simulink model "visual_line_follower_ppo_residual"  (R2026a)
settings: Solver=FixedStepDiscrete  StopTime=50  FixedStep=MJ_StepTime  EnableMultiTasking=on
InitFcn:
  | run(fullfile(fileparts(get_param(bdroot,"FileName")),"runtime","configure_turtlebot3_visual_line_follower_paths.m"));
model workspace (MAT data in the model file):
  BaseLinearSpeed = 20
  BaseSpeedScale = 0.03
  Kd_Line = 0.35
  Ki_Line = 0
  Kp_Line = 5
  LocalPath_CurvatureGain = 0.04
  LocalPath_HeadingGain = 0.35
  LocalPath_LateralGain = 0.6
  LocalPath_LookaheadDistance = 0.2
  LocalPath_NumPoints = 30
  LocalPath_ROIFraction = 0.5
  MJ_StepTime = 0.002
  MJ_TargetLateralPosition = 0
  MaxAngularSpeed = 1.5
  MaxWheelSpeed = 25
  N_Line = 20
  OriginBot_ErrorScale = 500
  OriginBot_MaxSaturation = 0.3
  OriginBot_MinBrightness = 70
  OriginBot_MinPixels = 30
  OriginBot_ROIHeight = 45
  OriginBot_ROIStartFraction = 0.72
  PPO_Done_Steps = 100
  PPO_MaxDeltaOmega = 1
  PPO_P_Lost = 10
  PPO_Q = 1
  PPO_R = 0.1
  SteeringSign = -1
  TB3_WheelRadius = 0.033
  TB3_WheelSeparation = 0.16
  Ts_Control = 0.05
  Ts_Stop = 10
  Ts_Vision = 0.05
  TurtleBot3MuJoCoMap = "track_hard"
  TurtleBot3MuJoCoScene = ""
undefined symbols (not defined in the file): originbot_line_follower_debug_frame, originbot_sliding_window_path_generator
libraries: mjLib x1, slpidlib x1, rllib x1
settings Model: ExtModeTrigDuration=10000  Creator=HP  LastModifiedBy=HP
settings SolverCC: PositivePriorityOrder=on
settings ConfigComp: CovMetricSettings=dswe

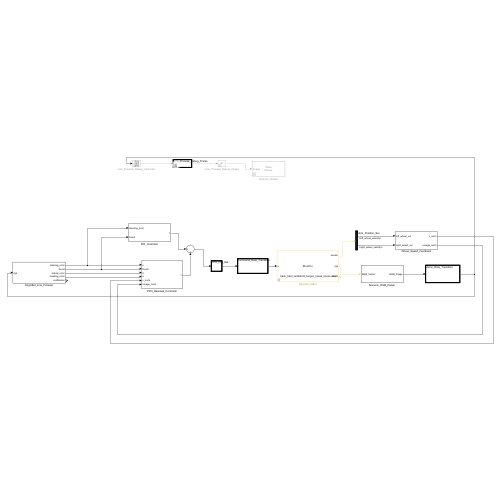
[thumbnail: Simulink's stored preview of the top-level diagram]
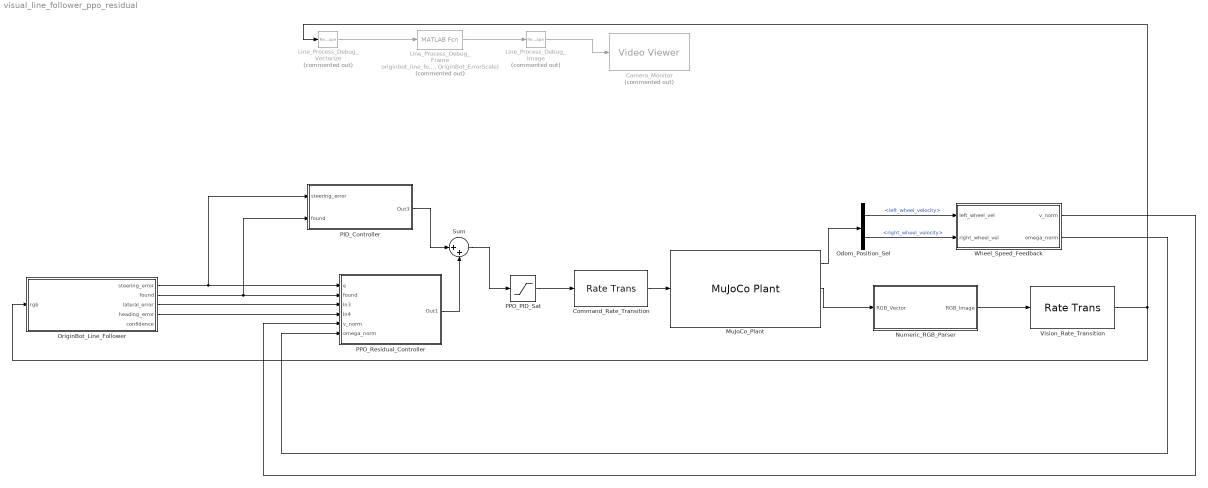
== system visual_line_follower_ppo_residual ==
  Camera_Monitor : VideoViewer  Commented=on  FigPos=[498 692 990 438]
  Command_Rate_Transition : RateTransition  OutPortSampleTime=MJ_StepTime
  Line_Process_Debug_Frame : MATLABFcn  Commented=on  MATLABFcn=originbot_line_follower_debug_frame(u, LocalPath_ROIFraction, LocalPath_NumPoints, OriginBot_MinBrightness, OriginBot_MaxSaturation, OriginBot_MinPixels, OriginBot_ErrorScale)
  Line_Process_Debug_Image : Reshape  Commented=on  OutputDimensionality=Customize  OutputDimensions=[480,640,3]
  Line_Process_Debug_Vectorize : Reshape  Commented=on  OutputDimensionality=Column vector (2-D)
  MuJoCo_Plant : mjLib/MuJoCo Plant  controlBus=[]  sensorBus=mj_bus_sensor_7979902499018342666  controlLength=[]  sensorLength=[]  rgbLength=[]  depthLength=[]  sampleTime=0.002  xmlFileRel=/media/kevin/ding/final_project/Sheffield/for_getting_started/src/simple_camera_pid/matlab/../../../model/mujoco/turtlebot3/track_hard_turtlebot3_burger_visual_scene.xml  xmlFile=/media/kevin/ding/final_project/Sheffield/for_getting_started/src/simple_camera_pid/matlab/../../../model/mujoco/turtlebot3/track_hard_turtlebot3_burger_visual_scene.xml  renderingType=None  vsync=on  visualFPS=60  zoomLevel=1  znear=0.062275  zfar=311.3772  cameraSampleTime=Ts_Vision  rgbOutOption=on  depthOutOption=off  controlInterfaceType=Vector
      settings: SourceProductName=MuJoCo Simulator
  Numeric_RGB_Parser : Subsystem
  Odom_Position_Sel : BusSelector  OutputSignals=left_wheel_velocity,right_wheel_velocity
  OriginBot_Line_Follower : Subsystem
  PID_Controller : Subsystem
  PPO_PID_Sat : Saturate  UpperLimit=[MaxWheelSpeed; MaxWheelSpeed]  LowerLimit=-[MaxWheelSpeed; MaxWheelSpeed]
  PPO_Residual_Controller : Subsystem
  Sum : Sum  Inputs=|++
  Vision_Rate_Transition : RateTransition  OutPortSampleTime=Ts_Vision
  Wheel_Speed_Feedback : Subsystem
  wires:
  Wheel_Speed_Feedback/2(omega_norm) -> PPO_Residual_Controller/6(omega_norm)
  Wheel_Speed_Feedback/1(v_norm) -> PPO_Residual_Controller/5(v_norm)
  Odom_Position_Sel/2 -> Wheel_Speed_Feedback/2(right_wheel_vel)  "<right_wheel_velocity>"
  Odom_Position_Sel/1 -> Wheel_Speed_Feedback/1(left_wheel_vel)  "<left_wheel_velocity>"
  Line_Process_Debug_Frame/1 -> Line_Process_Debug_Image/1
  Vision_Rate_Transition/1 -> OriginBot_Line_Follower/1(rgb), Line_Process_Debug_Vectorize/1
  Line_Process_Debug_Vectorize/1 -> Line_Process_Debug_Frame/1
  MuJoCo_Plant/2 -> Numeric_RGB_Parser/1(RGB_Vector)
  OriginBot_Line_Follower/2(found) -> PID_Controller/2(found), PPO_Residual_Controller/2(found)
  OriginBot_Line_Follower/1(steering_error) -> PID_Controller/1(steering_error), PPO_Residual_Controller/1(e)
  Command_Rate_Transition/1 -> MuJoCo_Plant/1
  Line_Process_Debug_Image/1 -> Camera_Monitor/1
  Numeric_RGB_Parser/1(RGB_Image) -> Vision_Rate_Transition/1
  OriginBot_Line_Follower/3(lateral_error) -> PPO_Residual_Controller/3(In3)
  OriginBot_Line_Follower/4(heading_error) -> PPO_Residual_Controller/4(In4)
  PID_Controller/1(Out3) -> Sum/1
  PPO_Residual_Controller/1(Out1) -> Sum/2
  Sum/1 -> PPO_PID_Sat/1
  PPO_PID_Sat/1 -> Command_Rate_Transition/1
  MuJoCo_Plant/1 -> Odom_Position_Sel/1

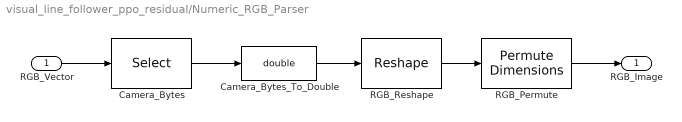
== system visual_line_follower_ppo_residual/Numeric_RGB_Parser ==
  RGB_Vector : Inport
  Camera_Bytes : Selector  InputPortWidth=921601  IndexOptions=Index vector (dialog)  Indices=1:921600  OutputSizes=1
  Camera_Bytes_To_Double : DataTypeConversion  OutDataTypeStr=double
  RGB_Permute : PermuteDimensions  Order=[3 2 1]
  RGB_Reshape : Reshape  OutputDimensionality=Customize  OutputDimensions=[3,640,480]
  RGB_Image : Outport
  wires:
  Camera_Bytes_To_Double/1 -> RGB_Reshape/1
  RGB_Permute/1 -> RGB_Image/1
  RGB_Reshape/1 -> RGB_Permute/1
  Camera_Bytes/1 -> Camera_Bytes_To_Double/1
  RGB_Vector/1 -> Camera_Bytes/1

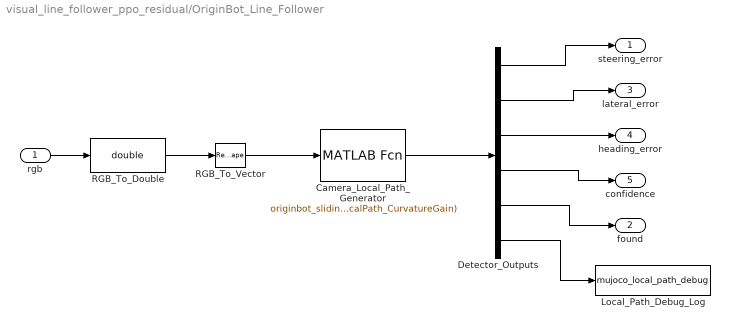
== system visual_line_follower_ppo_residual/OriginBot_Line_Follower ==
  rgb : Inport
  Camera_Local_Path_Generator : MATLABFcn  MATLABFcn=originbot_sliding_window_path_generator(u, LocalPath_ROIFraction, LocalPath_NumPoints, OriginBot_MinBrightness, OriginBot_MaxSaturation, OriginBot_MinPixels, OriginBot_ErrorScale, LocalPath_LookaheadDistance, LocalPath_LateralGain, LocalPath_HeadingGain, LocalPath_CurvatureGain)  OutputDimensions=72  OutputSignalType=real  SampleTime=Ts_Vision
  Detector_Outputs : Demux  Outputs=[1 1 1 1 1 67]
  Local_Path_Debug_Log : ToWorkspace  VariableName=mujoco_local_path_debug  SaveFormat=Timeseries  SampleTime=-1
  RGB_To_Double : DataTypeConversion  OutDataTypeStr=double
  RGB_To_Vector : Reshape  OutputDimensionality=Column vector (2-D)
  steering_error : Outport
  found : Outport  Port=2
  lateral_error : Outport  Port=3
  heading_error : Outport  Port=4
  confidence : Outport  Port=5
  wires:
  Detector_Outputs/2 -> lateral_error/1
  rgb/1 -> RGB_To_Double/1
  RGB_To_Double/1 -> RGB_To_Vector/1
  RGB_To_Vector/1 -> Camera_Local_Path_Generator/1
  Detector_Outputs/4 -> confidence/1
  Camera_Local_Path_Generator/1 -> Detector_Outputs/1
  Detector_Outputs/1 -> steering_error/1
  Detector_Outputs/3 -> heading_error/1
  Detector_Outputs/5 -> found/1
  Detector_Outputs/6 -> Local_Path_Debug_Log/1

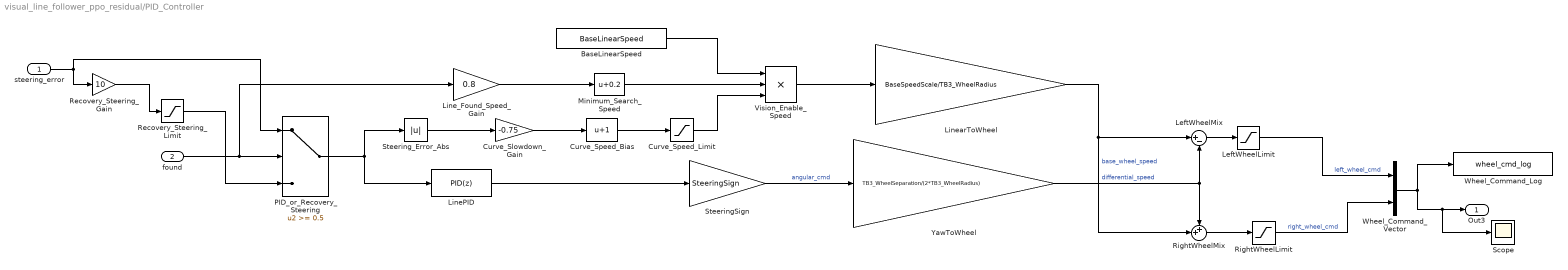
== system visual_line_follower_ppo_residual/PID_Controller ==
  steering_error : Inport
  found : Inport  Port=2
  BaseLinearSpeed : Constant  Value=BaseLinearSpeed
  Curve_Slowdown_Gain : Gain  Gain=-0.75
  Curve_Speed_Bias : Bias  Bias=1
  Curve_Speed_Limit : Saturate  UpperLimit=1  LowerLimit=0.25
  LeftWheelLimit : Saturate  UpperLimit=MaxWheelSpeed  LowerLimit=-MaxWheelSpeed
  LeftWheelMix : Sum  Inputs=|+-
  LinePID : slpidlib/PID Controller  Controller=PID  Form=Parallel  TimeDomain=Discrete-time  UseExternalTs=off  SampleTime=Ts_Control  IntegratorMethod=Backward Euler  FilterMethod=Trapezoidal  ControllerParametersSource=internal  P=Kp_Line  I=Ki_Line  UseKiTs=off  D=Kd_Line  UseExternalDerivativeSource=off  N=N_Line  UseFilter=on  TunerSelectOption=Transfer Function Based (PID Tuner App)  InitialConditionSource=internal  InitialConditionForIntegrator=0  InitialConditionForFilter=0  DifferentiatorICPrevScaledInput=0  ExternalReset=none  TrackingMode=off  Kt=1  LimitOutput=on  SatLimitsSource=internal  UpperSaturationLimit=MaxAngularSpeed  LowerSaturationLimit=-MaxAngularSpeed  LinearizeAsGain=off  AntiWindupMode=back-calculation  Kb=1  LimitIntegrator=off  UpperIntegratorSaturationLimit=inf  LowerIntegratorSaturationLimit=-inf  POutMin=[]  POutMax=[]  IOutMin=[]  IOutMax=[]  DOutMin=[]  DOutMax=[]  NOutMin=[]  NOutMax=[]  SumOutMin=[]  SumOutMax=[]  SaturationOutMin=[]  SaturationOutMax=[]  PParamMin=[]  PParamMax=[]  IParamMin=[]  IParamMax=[]  DParamMin=[]  DParamMax=[]  NParamMin=[]  NParamMax=[]  KbParamMin=[]  KbParamMax=[]  KtParamMin=[]  KtParamMax=[]  KbOutMin=[]  KbOutMax=[]  KtOutMin=[]  KtOutMax=[]  IntegratorOutMin=[]  IntegratorOutMax=[]  FilterOutMin=[]  FilterOutMax=[]  SumI1OutMin=[]  SumI1OutMax=[]  SumI2OutMin=[]  SumI2OutMax=[]  SumI3OutMin=[]  SumI3OutMax=[]  SumI4OutMin=[]  SumI4OutMax=[]  SumDOutMin=[]  SumDOutMax=[]  DifferentiatorOutMin=[]  DifferentiatorOutMax=[]  FilterDiffOutCoefMin=[]  FilterDiffOutCoefMax=[]  ReciprocalOutMin=[]  ReciprocalOutMax=[]  SumDenOutMin=[]  SumDenOutMax=[]  SumNumOutMin=[]  SumNumOutMax=[]  DivideOutMin=[]  DivideOutMax=[]  UdiffTsProdOutMin=[]  UdiffTsProdOutMax=[]  NTsProdOutMin=[]  NTsProdOutMax=[]  UintegralTsProdOutMin=[]  UintegralTsProdOutMax=[]  UngainTsProdOutMin=[]  UngainTsProdOutMax=[]  ClampingZeroOutDataTypeStr=Inherit: Inherit via back propagation  ClampingZeroOutMin=[]  ClampingZeroOutMax=[]  FilterDenConstantOutDataTypeStr=Inherit: Inherit via back propagation  FilterDenConstantOutMin=[]  FilterDenConstantOutMax=[]  PCopyOutDataTypeStr=Inherit: Inherit via back propagation  PCopyOutMin=[]  PCopyOutMax=[]  NCopyOutDataTypeStr=Inherit: Inherit via back propagation  NCopyOutMin=[]  NCopyOutMax=[]  IntegratorContinuousStateAttributes=''  IntegratorStateMustResolveToSignalObject=off  IntegratorRTWStateStorageClass=Auto  FilterContinuousStateAttributes=''  FilterStateMustResolveToSignalObject=off  FilterRTWStateStorageClass=Auto  ParallelPVariant=InternalParameters  IdealPVariant=Disabled  IVariant=InternalParameters  DVariant=InternalParameters  IntegratorVariant=Discrete  SatVariant=Enabled  AWVariant=BackCalculation  PCopyVariant=Disabled  TRVariant=Disabled  FdbkBlocksVariant=Feedback  IdealPFdbkVariant=Passthrough  SatFdbkVariant=Enabled  DerivativeFilterVariant=TrapezoidalFilter  NVariant=InternalParameters  NCopyVariant=InternalParameters  FilterICVariant=InternalICsFilter  IntegratorICVariant=InternalICs  ExternalResetVariant=Disabled  TRSumVariant=Passthrough  SumFdbkVariant=Enabled  SumVariant=Sum_PID  TsampFilterVariant=InternalTs  TsampNgainVariant=Passthrough  TsampIntegralVariant=Disabled_SignalSpec  ExternalSaturationOutDataTypeStr=Inherit: Same as second input  DerivativeSourceVariant=ErrorSignal  PreIntVariant=InternalPreInt
      settings: LibrarySourceBlock=hdlsllib/Discrete/Discrete PID Controller
  Line_Found_Speed_Gain : Gain  Gain=0.8
  LinearToWheel : Gain  Gain=BaseSpeedScale/TB3_WheelRadius
  Minimum_Search_Speed : Bias  Bias=0.2
  PID_or_Recovery_Steering : Switch  Threshold=0.5
  Recovery_Steering_Gain : Gain  Gain=10
  Recovery_Steering_Limit : Saturate  UpperLimit=0.45  LowerLimit=-0.45
  RightWheelLimit : Saturate  UpperLimit=MaxWheelSpeed  LowerLimit=-MaxWheelSpeed
  RightWheelMix : Sum  Inputs=++|
  Scope : Scope
  SteeringSign : Gain  Gain=SteeringSign
  Steering_Error_Abs : Abs
  Vision_Enable_Speed : Product  Inputs=***
  Wheel_Command_Log : ToWorkspace  VariableName=wheel_cmd_log  SaveFormat=Structure With Time
  Wheel_Command_Vector : Mux  Inputs=2
  YawToWheel : Gain  Gain=TB3_WheelSeparation/(2*TB3_WheelRadius)
  Out3 : Outport
  wires:
  LeftWheelLimit/1 -> Wheel_Command_Vector/1  "left_wheel_cmd"
  steering_error/1 -> Recovery_Steering_Gain/1, PID_or_Recovery_Steering/1
  Minimum_Search_Speed/1 -> Vision_Enable_Speed/2
  found/1 -> Line_Found_Speed_Gain/1, PID_or_Recovery_Steering/2
  PID_or_Recovery_Steering/1 -> Steering_Error_Abs/1, LinePID/1
  Recovery_Steering_Gain/1 -> Recovery_Steering_Limit/1
  Recovery_Steering_Limit/1 -> PID_or_Recovery_Steering/3
  Line_Found_Speed_Gain/1 -> Minimum_Search_Speed/1
  Steering_Error_Abs/1 -> Curve_Slowdown_Gain/1
  Curve_Slowdown_Gain/1 -> Curve_Speed_Bias/1
  Curve_Speed_Bias/1 -> Curve_Speed_Limit/1
  LinePID/1 -> SteeringSign/1
  BaseLinearSpeed/1 -> Vision_Enable_Speed/1
  Curve_Speed_Limit/1 -> Vision_Enable_Speed/3
  Vision_Enable_Speed/1 -> LinearToWheel/1
  SteeringSign/1 -> YawToWheel/1  "angular_cmd"
  LinearToWheel/1 -> LeftWheelMix/1, RightWheelMix/2  "base_wheel_speed"
  YawToWheel/1 -> RightWheelMix/1, LeftWheelMix/2  "differential_speed"
  LeftWheelMix/1 -> LeftWheelLimit/1
  RightWheelMix/1 -> RightWheelLimit/1
  RightWheelLimit/1 -> Wheel_Command_Vector/2  "right_wheel_cmd"
  Wheel_Command_Vector/1 -> Scope/1, Out3/1, Wheel_Command_Log/1

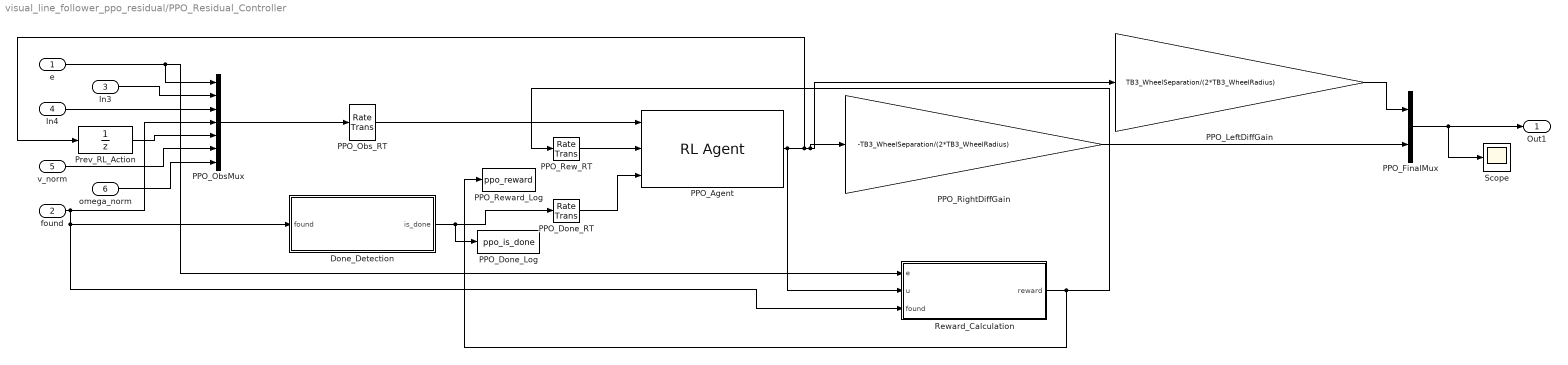
== system visual_line_follower_ppo_residual/PPO_Residual_Controller ==
  e : Inport
  found : Inport  Port=2
  In3 : Inport  Port=3
  In4 : Inport  Port=4
  v_norm : Inport  Port=5
  omega_norm : Inport  Port=6
  Done_Detection : Subsystem
  PPO_Agent : rllib/RL Agent  Agent=agent  ExternalActionAsInput=off  ProvideLastAction=off  ProvideCumRwd=off  TreatAsDirectFeedthrough=on  UseStrictObservationDataTypes=off
  PPO_Done_Log : ToWorkspace  VariableName=ppo_is_done  SaveFormat=Timeseries  SampleTime=-1
  PPO_Done_RT : RateTransition  Integrity=off  Deterministic=off
  PPO_FinalMux : Mux  Inputs=2
  PPO_LeftDiffGain : Gain  Gain=TB3_WheelSeparation/(2*TB3_WheelRadius)
  PPO_ObsMux : Mux  Inputs=7
  PPO_Obs_RT : RateTransition  Integrity=off  Deterministic=off
  PPO_Rew_RT : RateTransition  Integrity=off  Deterministic=off
  PPO_Reward_Log : ToWorkspace  VariableName=ppo_reward  SaveFormat=Timeseries  SampleTime=-1
  PPO_RightDiffGain : Gain  Gain=-TB3_WheelSeparation/(2*TB3_WheelRadius)
  Prev_RL_Action : UnitDelay  SampleTime=Ts_Control
  Reward_Calculation : Subsystem
  Scope : Scope
      settings: ActiveDisplayYMinimum=-1  ActiveDisplayYMaximum=1
  Out1 : Outport
  wires:
  omega_norm/1 -> PPO_ObsMux/7
  v_norm/1 -> PPO_ObsMux/6
  Done_Detection/1(is_done) -> PPO_Done_RT/1, PPO_Done_Log/1
  Reward_Calculation/1(reward) -> PPO_Reward_Log/1, PPO_Rew_RT/1
  PPO_FinalMux/1 -> Out1/1, Scope/1
  PPO_RightDiffGain/1 -> PPO_FinalMux/2
  PPO_LeftDiffGain/1 -> PPO_FinalMux/1
  PPO_ObsMux/1 -> PPO_Obs_RT/1
  Prev_RL_Action/1 -> PPO_ObsMux/5
  In4/1 -> PPO_ObsMux/3
  In3/1 -> PPO_ObsMux/2
  PPO_Agent/1 -> PPO_LeftDiffGain/1, PPO_RightDiffGain/1, Prev_RL_Action/1, Reward_Calculation/2(u)
  PPO_Obs_RT/1 -> PPO_Agent/1
  PPO_Done_RT/1 -> PPO_Agent/3
  PPO_Rew_RT/1 -> PPO_Agent/2
  found/1 -> Reward_Calculation/3(found), Done_Detection/1(found), PPO_ObsMux/4
  e/1 -> Reward_Calculation/1(e), PPO_ObsMux/1

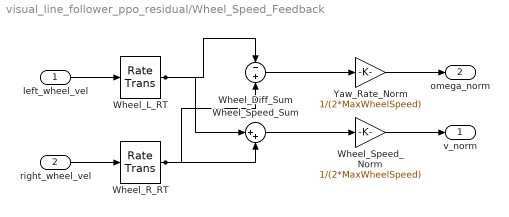
== system visual_line_follower_ppo_residual/Wheel_Speed_Feedback ==
  left_wheel_vel : Inport
  right_wheel_vel : Inport  Port=2
  Wheel_Diff_Sum : Sum  Inputs=-+
  Wheel_L_RT : RateTransition  OutPortSampleTime=Ts_Control
  Wheel_R_RT : RateTransition  OutPortSampleTime=Ts_Control
  Wheel_Speed_Norm : Gain  Gain=1/(2*MaxWheelSpeed)
  Wheel_Speed_Sum : Sum  Inputs=|++
  Yaw_Rate_Norm : Gain  Gain=1/(2*MaxWheelSpeed)
  v_norm : Outport
  omega_norm : Outport  Port=2
  wires:
  Yaw_Rate_Norm/1 -> omega_norm/1
  Wheel_Speed_Norm/1 -> v_norm/1
  Wheel_Diff_Sum/1 -> Yaw_Rate_Norm/1
  Wheel_Speed_Sum/1 -> Wheel_Speed_Norm/1
  Wheel_R_RT/1 -> Wheel_Speed_Sum/2, Wheel_Diff_Sum/2
  Wheel_L_RT/1 -> Wheel_Speed_Sum/1, Wheel_Diff_Sum/1
  right_wheel_vel/1 -> Wheel_R_RT/1
  left_wheel_vel/1 -> Wheel_L_RT/1

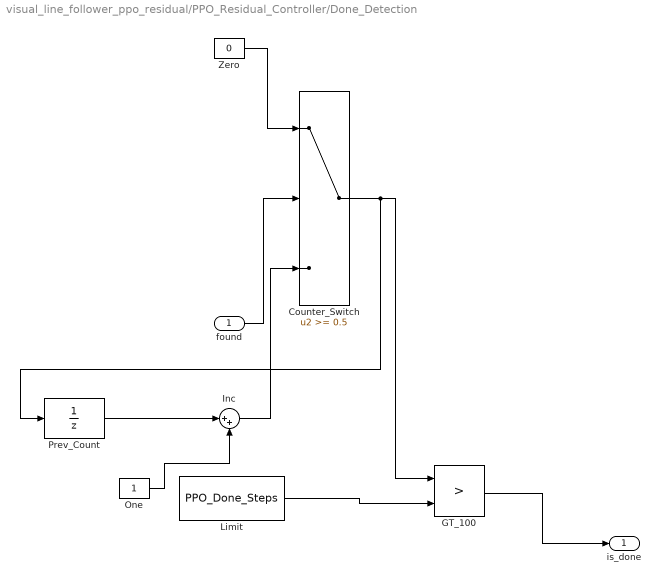
== system visual_line_follower_ppo_residual/PPO_Residual_Controller/Done_Detection ==
  found : Inport
  Counter_Switch : Switch  Threshold=0.5  SaturateOnIntegerOverflow=off  InputSameDT=off
  GT_100 : RelationalOperator  Operator=>  OutDataTypeStr=boolean  RndMeth=Simplest  InputSameDT=off
  Inc : Sum  Inputs=|++
  Limit : Constant  Value=PPO_Done_Steps
  One : Constant
  Prev_Count : UnitDelay  SampleTime=Ts_Control
  Zero : Constant  Value=0
  is_done : Outport
  wires:
  Counter_Switch/1 -> GT_100/1, Prev_Count/1
  Limit/1 -> GT_100/2
  Inc/1 -> Counter_Switch/3
  Zero/1 -> Counter_Switch/1
  found/1 -> Counter_Switch/2
  One/1 -> Inc/2
  Prev_Count/1 -> Inc/1
  GT_100/1 -> is_done/1

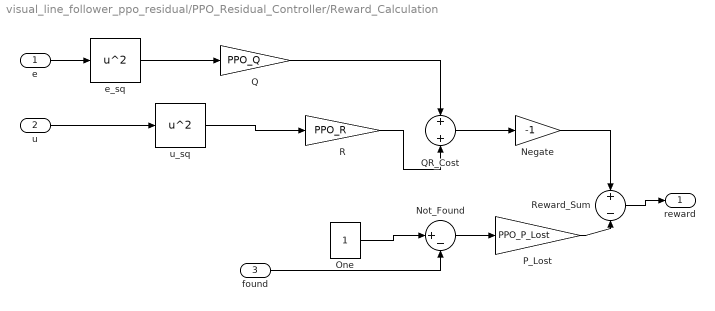
== system visual_line_follower_ppo_residual/PPO_Residual_Controller/Reward_Calculation ==
  e : Inport
  u : Inport  Port=2
  found : Inport  Port=3
  Negate : Gain  Gain=-1
  Not_Found : Sum  Inputs=|+-
  One : Constant
  P_Lost : Gain  Gain=PPO_P_Lost
  Q : Gain  Gain=PPO_Q
  QR_Cost : Sum
  R : Gain  Gain=PPO_R
  Reward_Sum : Sum  Inputs=+-
  e_sq : Math  Operator=square
  u_sq : Math  Operator=square
  reward : Outport
  wires:
  Reward_Sum/1 -> reward/1
  Negate/1 -> Reward_Sum/1
  P_Lost/1 -> Reward_Sum/2
  Not_Found/1 -> P_Lost/1
  QR_Cost/1 -> Negate/1
  found/1 -> Not_Found/2
  One/1 -> Not_Found/1
  u_sq/1 -> R/1
  e_sq/1 -> Q/1
  R/1 -> QR_Cost/2
  u/1 -> u_sq/1
  e/1 -> e_sq/1
  Q/1 -> QR_Cost/1
